simulink model "NonLinearHinf"  (R2021a)
settings: Solver=VariableStepAuto  StartTime=0.0  StopTime=10.0  RelTol=1e-3
values from neighbouring files (symbols this model uses):
  A = [0 0 1 0 ... (first row only)    [HeliControlGain.m]    (also in HeliControlHinf.m; HeliControlInteger.m; HeliControlLQG.m; HeliControlLQRgain.m)
  B = [0 0 ... (first row only)    [HeliControlGain.m]    (also in HeliControlHinf.m; HeliControlInteger.m; HeliControlLQG.m; HeliControlLQRgain.m)
  Bp = 0.8    [HeliControlGain.m]    (also in HeliControlHinf.m; HeliControlInteger.m; HeliControlIntegerObsv.m; HeliControlLQG.m)
  By = 0.318    [HeliControlGain.m]    (also in HeliControlHinf.m; HeliControlInteger.m; HeliControlIntegerObsv.m; HeliControlLQG.m)
  C = [1 0 0 0 ... (first row only)    [HeliControlGain.m]    (also in HeliControlHinf.m; HeliControlInteger.m; HeliControlLQG.m; HeliControlLQRgain.m)
  D = zeros(2,2)    [HeliControlGain.m]    (also in HeliControlHinf.m; HeliControlInteger.m; HeliControlLQG.m; HeliControlLQRgain.m)
  g = 9.81    [HeliControlGain.m]    (also in HeliControlHinf.m; HeliControlInteger.m; HeliControlIntegerObsv.m; HeliControlLQG.m)
  Jeq_y = 0.0432    [HeliControlGain.m]    (also in HeliControlHinf.m; HeliControlInteger.m; HeliControlIntegerObsv.m; HeliControlLQG.m)
  Jtp = Jeq_p + Mheli*Lcm^2    (= 0.0863915712)    [HeliControlGain.m]    (also in HeliControlHinf.m; HeliControlInteger.m; HeliControlIntegerObsv.m; HeliControlLQG.m)
  Kpp = 0.204    [HeliControlGain.m]    (also in HeliControlHinf.m; HeliControlInteger.m; HeliControlIntegerObsv.m; HeliControlLQG.m)
  Kpy = 0.0068    [HeliControlGain.m]    (also in HeliControlHinf.m; HeliControlInteger.m; HeliControlIntegerObsv.m; HeliControlLQG.m)
  Kyp = 0.0219    [HeliControlGain.m]    (also in HeliControlHinf.m; HeliControlInteger.m; HeliControlIntegerObsv.m; HeliControlLQG.m)
  Kyy = 0.072    [HeliControlGain.m]    (also in HeliControlHinf.m; HeliControlInteger.m; HeliControlIntegerObsv.m; HeliControlLQG.m)
  Lcm = 0.186    [HeliControlGain.m]    (also in HeliControlHinf.m; HeliControlInteger.m; HeliControlIntegerObsv.m; HeliControlLQG.m)
  Mheli = 1.3872    [HeliControlGain.m]    (also in HeliControlHinf.m; HeliControlInteger.m; HeliControlIntegerObsv.m; HeliControlLQG.m)
  u0 = a\b    [HeliControlGain.m]    (also in HeliControlHinf.m; HeliControlInteger.m; HeliControlIntegerObsv.m; HeliControlLQG.m)
libraries: simulink x6, cstblocks x2
settings Model: Creator=Ciro  LastModifiedBy=Ciro

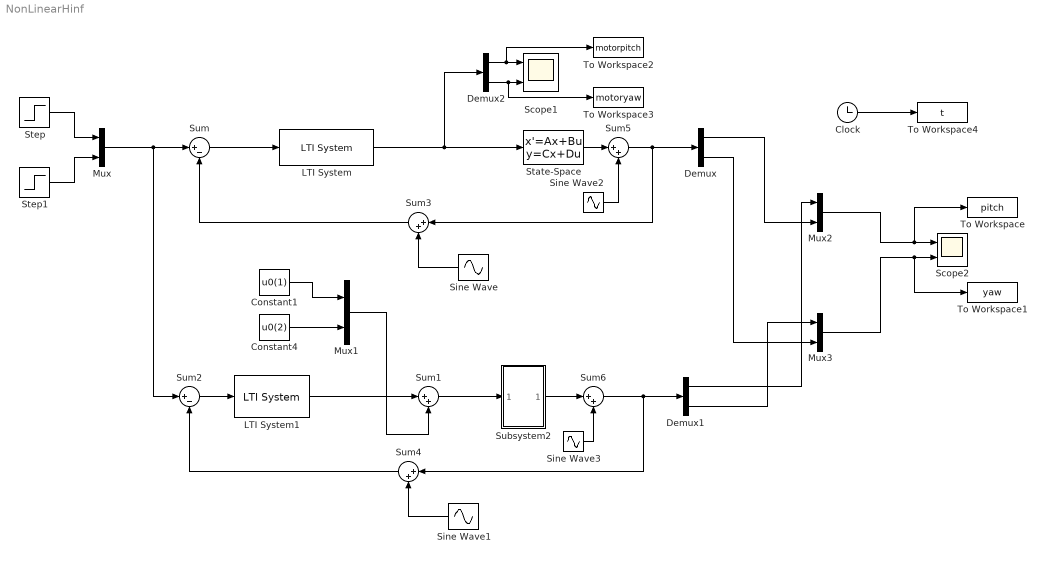
== system NonLinearHinf ==
  Clock : Clock
  Constant1 : Constant  Value=u0(1)
  Constant4 : Constant  Value=u0(2)
  Demux : Demux  Outputs=2
  Demux1 : Demux  Outputs=2
  Demux2 : Demux  Outputs=2
  LTI System : cstblocks/LTI System  sys=K  IC=[]
  LTI System1 : cstblocks/LTI System  sys=K  IC=[]
  Mux{,1..3} (4 alike) : Mux  Inputs=2
  Scope1 : Scope  NumInputPorts=2
  Scope2 : Scope  NumInputPorts=2
  Sine Wave : Sin  Amplitude=0  Frequency=100  SampleTime=0
  Sine Wave1 : Sin  Amplitude=0  Frequency=100  SampleTime=0
  Sine Wave2 : Sin  Amplitude=0  Frequency=1e-4  SampleTime=0
  Sine Wave3 : Sin  Amplitude=0  Frequency=1e-4  SampleTime=0
  State-Space : StateSpace  A=A  B=B  C=C  D=D  InitialCondition=[0;0;0;0]
  Step : Step  After=0.3  SampleTime=0
  Step1 : Step  After=0.3  SampleTime=0
  Subsystem2 : Subsystem
  Sum : Sum  Inputs=|+-
  Sum{1,3..6} (5 alike) : Sum  Inputs=|++
  Sum2 : Sum  Inputs=|+-
  To Workspace : ToWorkspace  VariableName=pitch  SampleTime=-1
      settings: Save2DSignal=2-D array (concatenate along first dimension)
  To Workspace1 : ToWorkspace  VariableName=yaw  SampleTime=-1
      settings: Save2DSignal=2-D array (concatenate along first dimension)
  To Workspace2 : ToWorkspace  VariableName=motorpitch  SampleTime=-1
      settings: Save2DSignal=2-D array (concatenate along first dimension)
  To Workspace3 : ToWorkspace  VariableName=motoryaw  SampleTime=-1
      settings: Save2DSignal=2-D array (concatenate along first dimension)
  To Workspace4 : ToWorkspace  VariableName=t  SampleTime=-1
      settings: Save2DSignal=2-D array (concatenate along first dimension)
  wires:
  Sum/1 -> LTI System/1
  Sum1/1 -> Subsystem2/1(In1)
  Demux/1 -> Mux2/2
  Demux1/1 -> Mux2/1
  Demux1/2 -> Mux3/1
  Mux2/1 -> To Workspace/1, Scope2/1
  Mux3/1 -> To Workspace1/1, Scope2/2
  Subsystem2/1(Out1) -> Sum6/1
  State-Space/1 -> Sum5/1
  Constant4/1 -> Mux1/2
  Sum2/1 -> LTI System1/1
  Step/1 -> Mux/1
  Mux1/1 -> Sum1/2
  Constant1/1 -> Mux1/1
  Demux/2 -> Mux3/2
  LTI System/1 -> Demux2/1, State-Space/1
  Mux/1 -> Sum2/1, Sum/1
  LTI System1/1 -> Sum1/1
  Step1/1 -> Mux/2
  Sum3/1 -> Sum/2
  Sine Wave/1 -> Sum3/2
  Sine Wave1/1 -> Sum4/2
  Sum4/1 -> Sum2/2
  Sum5/1 -> Sum3/1, Demux/1
  Sine Wave2/1 -> Sum5/2
  Sum6/1 -> Sum4/1, Demux1/1
  Sine Wave3/1 -> Sum6/2
  Demux2/1 -> To Workspace2/1, Scope1/1
  Demux2/2 -> To Workspace3/1, Scope1/2
  Clock/1 -> To Workspace4/1

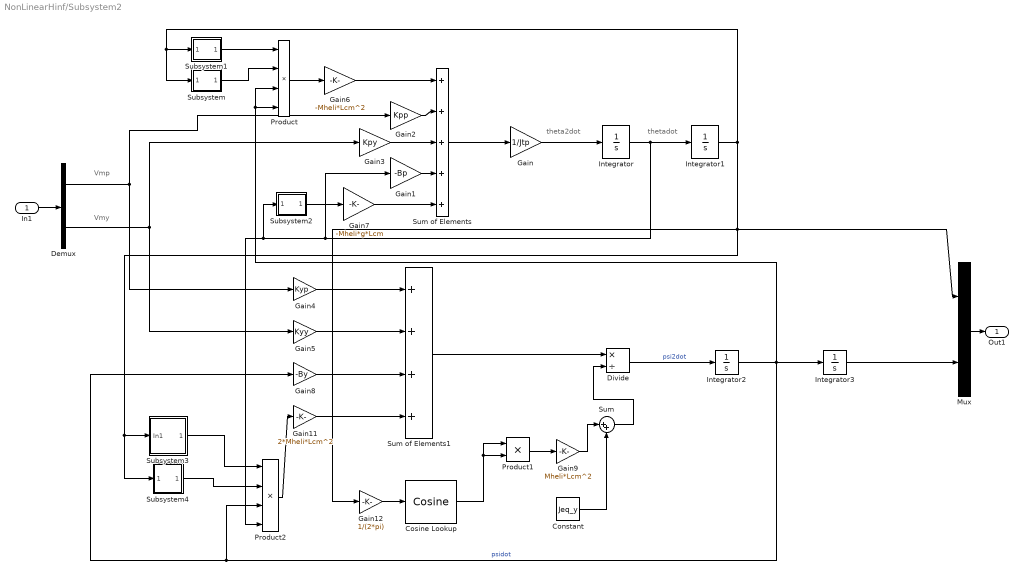
== system NonLinearHinf/Subsystem2 ==
  note: theta2dot
  note: thetadot
  note: Vmy
  note: Vmp
  In1 : Inport
  Constant : Constant  Value=Jeq_y
  Cosine Lookup : simulink/Lookup Tables/Cosine  Formula=cos(2*pi*u)  NumDataPoints=(2^5)+1  OutputWordLength=16  InternalRulePriority=Speed
      settings: SourceProductBaseCode=SL
  Demux : Demux  Outputs=2
  Divide : Product  Inputs=*/
  Gain : Gain  Gain=1/Jtp
  Gain1 : Gain  Gain=-Bp
  Gain11 : Gain  Gain=2*Mheli*Lcm^2
  Gain12 : Gain  Gain=1/(2*pi)
  Gain2 : Gain  Gain=Kpp
  Gain3 : Gain  Gain=Kpy
  Gain4 : Gain  Gain=Kyp
  Gain5 : Gain  Gain=Kyy
  Gain6 : Gain  Gain=-Mheli*Lcm^2
  Gain7 : Gain  Gain=-Mheli*g*Lcm
  Gain8 : Gain  Gain=-By
  Gain9 : Gain  Gain=Mheli*Lcm^2
  Integrator{,1..3} (4 alike) : Integrator
  Mux : Mux  Inputs=2
  Product : Product  Inputs=4
  Product1 : Product
  Product2 : Product  Inputs=4
  Subsystem : Subsystem
  Subsystem1 : Subsystem
  Subsystem2 : Subsystem
  Subsystem3 : Subsystem
  Subsystem4 : Subsystem
  Sum : Sum  Inputs=|++
  Sum of Elements : Sum  Inputs=+++++
  Sum of Elements1 : Sum  Inputs=++++
  Out1 : Outport
  wires:
  Gain5/1 -> Sum of Elements1/2
  Gain9/1 -> Sum/1
  In1/1 -> Demux/1
  Product1/1 -> Gain9/1
  Subsystem1/1(sin(2*pi*u)) -> Product/1
  Gain3/1 -> Sum of Elements/3
  Gain6/1 -> Sum of Elements/1
  Subsystem/1(cos(2*pi*u)) -> Product/2
  Constant/1 -> Sum/2
  Subsystem4/1(sin(2*pi*u)) -> Product2/2
  Gain12/1 -> Cosine Lookup/1
  Gain2/1 -> Sum of Elements/2
  Sum of Elements1/1 -> Divide/1
  Cosine Lookup/1 -> Product1/1, Product1/2
  Gain11/1 -> Sum of Elements1/4
  Mux/1 -> Out1/1
  Gain4/1 -> Sum of Elements1/1
  Gain8/1 -> Sum of Elements1/3
  Product/1 -> Gain6/1
  Gain7/1 -> Sum of Elements/5
  Integrator3/1 -> Mux/2
  Demux/1 -> Gain2/1, Gain4/1
  Demux/2 -> Gain3/1, Gain5/1
  Subsystem2/1(cos(2*pi*u)) -> Gain7/1
  Integrator2/1 -> Integrator3/1, Product2/3, Gain8/1, Product/3, Product/4  "psidot"
  Sum/1 -> Divide/2
  Sum of Elements/1 -> Gain/1
  Gain1/1 -> Sum of Elements/4
  Integrator1/1 -> Subsystem1/1(In1), Subsystem/1(In1), Gain12/1, Mux/1, Subsystem3/1(In1), Subsystem4/1(In1)
  Product2/1 -> Gain11/1
  Subsystem3/1(cos(2*pi*u)) -> Product2/1
  Integrator/1 -> Integrator1/1, Subsystem2/1(In1), Product2/4, Gain1/1
  Gain/1 -> Integrator/1
  Divide/1 -> Integrator2/1  "psi2dot"

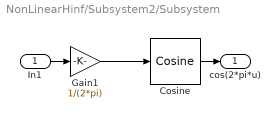
== system NonLinearHinf/Subsystem2/Subsystem ==
  In1 : Inport
  Cosine : simulink/Lookup Tables/Cosine  Formula=cos(2*pi*u)  NumDataPoints=(2^5)+1  OutputWordLength=16  InternalRulePriority=Speed
      settings: SourceProductBaseCode=SL
  Gain1 : Gain  Gain=1/(2*pi)
  cos(2*pi*u) : Outport
  wires:
  Cosine/1 -> cos(2*pi*u)/1
  In1/1 -> Gain1/1
  Gain1/1 -> Cosine/1

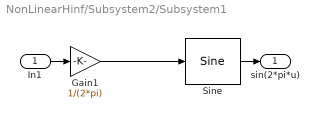
== system NonLinearHinf/Subsystem2/Subsystem1 ==
  In1 : Inport
  Gain1 : Gain  Gain=1/(2*pi)
  Sine : simulink/Lookup Tables/Sine  Formula=sin(2*pi*u)  NumDataPoints=(2^5)+1  OutputWordLength=16  InternalRulePriority=Speed
  sin(2*pi*u) : Outport
  wires:
  Sine/1 -> sin(2*pi*u)/1
  In1/1 -> Gain1/1
  Gain1/1 -> Sine/1

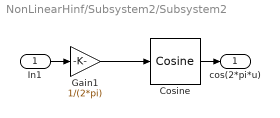
== system NonLinearHinf/Subsystem2/Subsystem2 ==
  In1 : Inport
  Cosine : simulink/Lookup Tables/Cosine  Formula=cos(2*pi*u)  NumDataPoints=(2^5)+1  OutputWordLength=16  InternalRulePriority=Speed
      settings: SourceProductBaseCode=SL
  Gain1 : Gain  Gain=1/(2*pi)
  cos(2*pi*u) : Outport
  wires:
  Gain1/1 -> Cosine/1
  In1/1 -> Gain1/1
  Cosine/1 -> cos(2*pi*u)/1

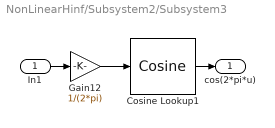
== system NonLinearHinf/Subsystem2/Subsystem3 ==
  In1 : Inport
  Cosine Lookup1 : simulink/Lookup Tables/Cosine  Formula=cos(2*pi*u)  NumDataPoints=(2^5)+1  OutputWordLength=16  InternalRulePriority=Speed
      settings: SourceProductBaseCode=SL
  Gain12 : Gain  Gain=1/(2*pi)
  cos(2*pi*u) : Outport
  wires:
  Cosine Lookup1/1 -> cos(2*pi*u)/1
  In1/1 -> Gain12/1
  Gain12/1 -> Cosine Lookup1/1

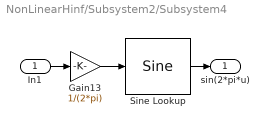
== system NonLinearHinf/Subsystem2/Subsystem4 ==
  In1 : Inport
  Gain13 : Gain  Gain=1/(2*pi)
  Sine Lookup : simulink/Lookup Tables/Sine  Formula=sin(2*pi*u)  NumDataPoints=(2^5)+1  OutputWordLength=16  InternalRulePriority=Speed
  sin(2*pi*u) : Outport
  wires:
  In1/1 -> Gain13/1
  Sine Lookup/1 -> sin(2*pi*u)/1
  Gain13/1 -> Sine Lookup/1
